simulink model "LCA_feature_mode"  (R2021a)
settings: Solver=VariableStepAuto  StartTime=0.0  StopTime=sim_time  RelTol=1e-3
values from neighbouring files (symbols this model uses):
  L = 4.7    [Pure_Pursiut_Controller_init.m]    (also in Stanley_control_init.m)
  Ld = 10    [Pure_Pursiut_Controller_init.m]
  Vx = 25    [mpc_init.m]
  xRef = refpose(1,:)    [Stanley_control_init.m]    (also in mpc_init.m = refPose(1,:))
  yRef = refpose(2,:)    [Stanley_control_init.m]    (also in mpc_init.m = refPose(2,:) + 2)
undefined symbols (not defined in the file or in its folder): sigbuilder_block
libraries: simulink x2, robotalgslib x1
settings Model: Creator=User  LastModifiedBy=User

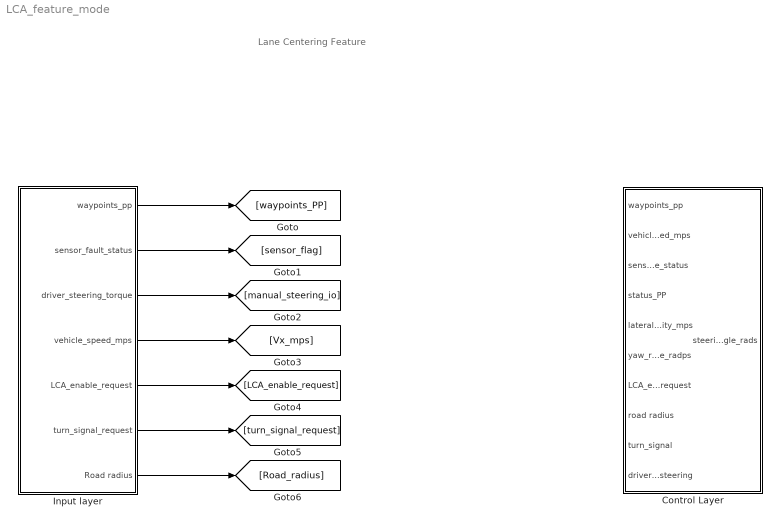
== system LCA_feature_mode ==
  note: Lane Centering Feature
  "\tControl Layer" : Subsystem
  Input layer : Subsystem
  wires:
  Input layer/1(waypoints_pp) -> [waypoints_PP]
  Input layer/2(sensor_fault_status) -> [sensor_flag]
  Input layer/3(driver_steering_torque) -> [manual_steering_io]
  Input layer/4(vehicle_speed_mps) -> [Vx_mps]
  Input layer/5(LCA_enable_request) -> [LCA_enable_request]
  Input layer/6(turn_signal_request) -> [turn_signal_request]
  Input layer/7(Road radius) -> [Road_radius]

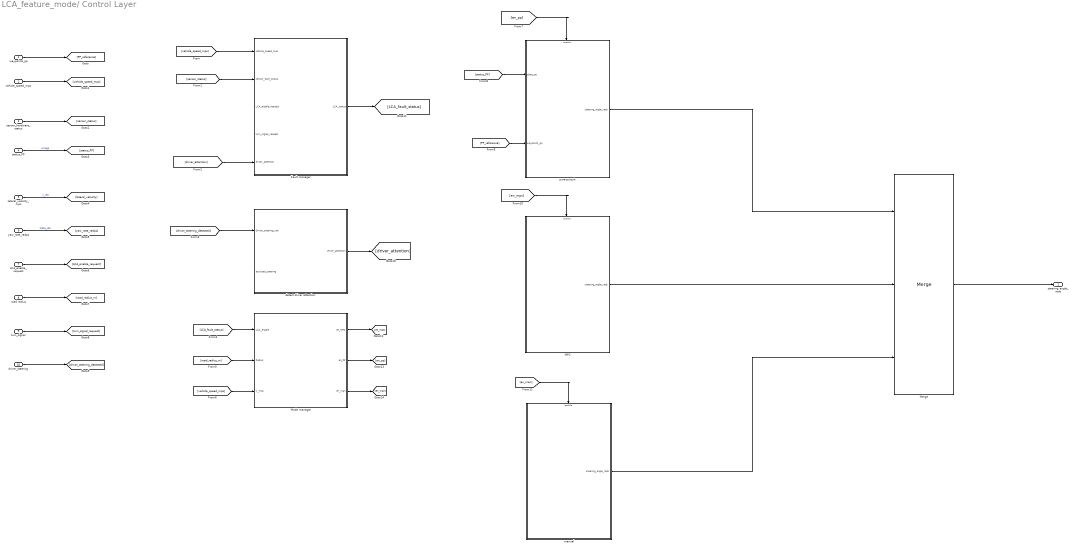
== system LCA_feature_mode/	Control Layer ==
  waypoints_pp : Inport
  vehicle_speed_mps : Inport  Port=2
  sensor_hardware_status : Inport  Port=3
  status_PP : Inport  Port=4
  lateral_velocity_mps : Inport  Port=5
  yaw_rate_radps : Inport  Port=6
  LCA_enable_request : Inport  Port=7
  road radius : Inport  Port=8
  turn_signal : Inport  Port=9
  driver_steering : Inport  Port=10
  Fault manager : Subsystem
  MPC : Subsystem
  Merge : Merge  Inputs=3
  Mode manager : Subsystem
  detect driver attention : Subsystem
  manual : Subsystem
  pure-pursuit : Subsystem
  steering_angle_rads : Outport
  wires:
  waypoints_pp/1 -> [PP_reference]
  vehicle_speed_mps/1 -> [vehicle_speed_mps]
  sensor_hardware_status/1 -> [sensor_status]
  status_PP/1 -> [status_PP]  "omega"
  lateral_velocity_mps/1 -> [lateral_velocity]  "y_dot"
  yaw_rate_radps/1 -> [yaw_rate_radps]  "theta_dot"
  LCA_enable_request/1 -> [LCA_enable_request]
  road radius/1 -> [road_radius_m]
  turn_signal/1 -> [turn_signal_request]
  driver_steering/1 -> [driver_steering_detected]
  [vehicle_speed_mps] -> Fault manager/1(vehicle_speed_mps)
  [sensor_status] -> Fault manager/2(sensor_fault_status)
  detect driver attention/1(driver_attention) -> [driver_attention]
  [driver_attention] -> Fault manager/5("\tdriver_attention")
  [driver_steering_detected] -> detect driver attention/1(Driver_steering_rad)
  Fault manager/1(LCA_status) -> [LCA_fault_status]
  [LCA_fault_status] -> Mode manager/1(LCA_enable)
  [road_radius_m] -> Mode manager/2(Radius)
  [vehicle_speed_mps] -> Mode manager/3(V_mps)
  Mode manager/1(en_MPC) -> [en_mpc]
  Mode manager/2(en_PP) -> [en_pp]
  Mode manager/3(en_man) -> [en_man]
  [en_pp] -> pure-pursuit/Enable
  [status_PP] -> pure-pursuit/1(state_pp)
  [PP_reference] -> pure-pursuit/2(waypoints_pp)
  pure-pursuit/1(steering_angle_rads) -> Merge/1
  MPC/1(steering_angle_rads) -> Merge/2
  [en_mpc] -> MPC/Enable
  [en_man] -> manual/Enable
  manual/1(steering_angle_rads) -> Merge/3
  Merge/1 -> steering_angle_rads/1

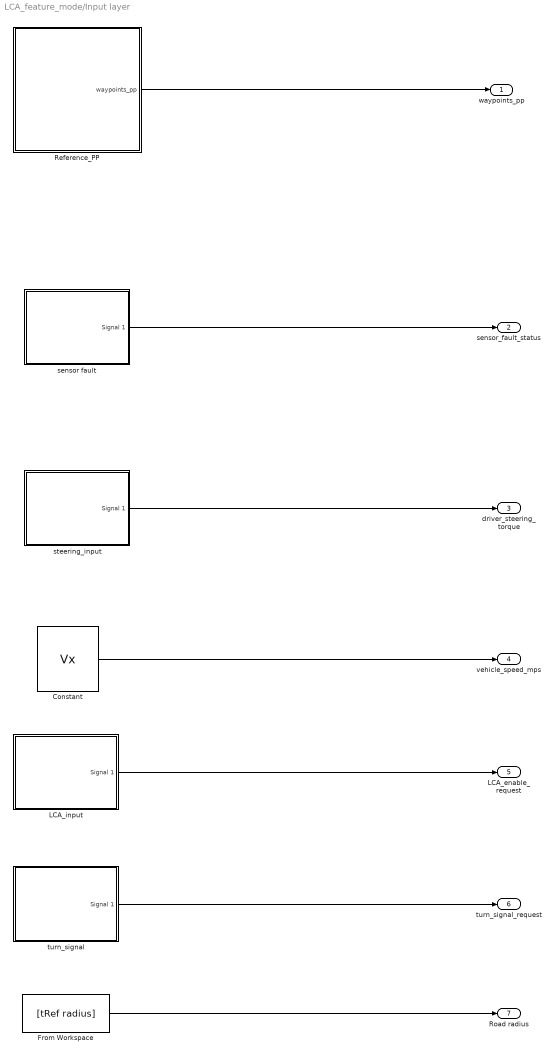
== system LCA_feature_mode/Input layer ==
  Constant : Constant  Value=Vx
  From Workspace : FromWorkspace  VariableName=[tRef radius]  SampleTime=0.1
  LCA_input : Subsystem  Tag=STV Subsys  LoadFcn=sigbuilder_block('load');  StartFcn=sigbuilder_block('start');  StopFcn=sigbuilder_block('stop');  ClipboardFcn=sigbuilder_block('clipboard');  mask(Sigbuilder block){tuvar=[0:10]}
      mask help: Simulink:masks:SigbuilderBlock_MD
      mask init:
      | if ~strcmp(get_param(bdroot(gcbh),'SimulationStatus'),'stopped') tuvar = sigbuilder_block('maskInit'); end
      settings: CopyFcn=sigbuilder_block('copy');  DeleteFcn=sigbuilder_block('delete');  ModelCloseFcn=sigbuilder_block('modelClose');  PreSaveFcn=sigbuilder_block('preSave');  PauseFcn=sigbuilder_block('pause');  ContinueFcn=sigbuilder_block('continue');  NameChangeFcn=sigbuilder_block('namechange');  OpenFcn=sigbuilder_block('open',[309 216.75 550.5 359.25 ]);  CloseFcn=sigbuilder_block('close');
      mask Display: plot(0, 0, 100, 100,[2, 2, 32, 32, 2], [68, 8, 8, 68, 68],[32, 2], [38, 38], [32, 19, 2],[53, 60, 44], [32, 17, 17, 2],[16, 16, 31, 31]);txt = getActiveGroup(gcbh);text(2, 100, txt,'verticalAlignment', 'top');
  Reference_PP : Subsystem
  sensor fault : Subsystem  Tag=STV Subsys  LoadFcn=sigbuilder_block('load');  StartFcn=sigbuilder_block('start');  StopFcn=sigbuilder_block('stop');  ClipboardFcn=sigbuilder_block('clipboard');  mask(Sigbuilder block){tuvar=[0:10]}
      mask help: Simulink:masks:SigbuilderBlock_MD
      mask init:
      | if ~strcmp(get_param(bdroot(gcbh),'SimulationStatus'),'stopped') tuvar = sigbuilder_block('maskInit'); end
      settings: CopyFcn=sigbuilder_block('copy');  DeleteFcn=sigbuilder_block('delete');  ModelCloseFcn=sigbuilder_block('modelClose');  PreSaveFcn=sigbuilder_block('preSave');  PauseFcn=sigbuilder_block('pause');  ContinueFcn=sigbuilder_block('continue');  NameChangeFcn=sigbuilder_block('namechange');  OpenFcn=sigbuilder_block('open',[309 216.75 550.5 359.25 ]);  CloseFcn=sigbuilder_block('close');
      mask Display: plot(0, 0, 100, 100,[2, 2, 32, 32, 2], [68, 8, 8, 68, 68],[32, 2], [38, 38], [32, 19, 2],[53, 60, 44], [32, 17, 17, 2],[16, 16, 31, 31]);txt = getActiveGroup(gcbh);text(2, 100, txt,'verticalAlignment', 'top');
  steering_input : Subsystem  Tag=STV Subsys  LoadFcn=sigbuilder_block('load');  StartFcn=sigbuilder_block('start');  StopFcn=sigbuilder_block('stop');  ClipboardFcn=sigbuilder_block('clipboard');  mask(Sigbuilder block){tuvar=[0:10]}
      mask help: Simulink:masks:SigbuilderBlock_MD
      mask init:
      | if ~strcmp(get_param(bdroot(gcbh),'SimulationStatus'),'stopped') tuvar = sigbuilder_block('maskInit'); end
      settings: CopyFcn=sigbuilder_block('copy');  DeleteFcn=sigbuilder_block('delete');  ModelCloseFcn=sigbuilder_block('modelClose');  PreSaveFcn=sigbuilder_block('preSave');  PauseFcn=sigbuilder_block('pause');  ContinueFcn=sigbuilder_block('continue');  NameChangeFcn=sigbuilder_block('namechange');  OpenFcn=sigbuilder_block('open',[309 216.75 550.5 359.25 ]);  CloseFcn=sigbuilder_block('close');
      mask Display: plot(0, 0, 100, 100,[2, 2, 32, 32, 2], [68, 8, 8, 68, 68],[32, 2], [38, 38], [32, 19, 2],[53, 60, 44], [32, 17, 17, 2],[16, 16, 31, 31]);txt = getActiveGroup(gcbh);text(2, 100, txt,'verticalAlignment', 'top');
  turn_signal : Subsystem  Tag=STV Subsys  LoadFcn=sigbuilder_block('load');  StartFcn=sigbuilder_block('start');  StopFcn=sigbuilder_block('stop');  ClipboardFcn=sigbuilder_block('clipboard');  mask(Sigbuilder block){tuvar=[0:10]}
      mask help: Simulink:masks:SigbuilderBlock_MD
      mask init:
      | if ~strcmp(get_param(bdroot(gcbh),'SimulationStatus'),'stopped') tuvar = sigbuilder_block('maskInit'); end
      settings: CopyFcn=sigbuilder_block('copy');  DeleteFcn=sigbuilder_block('delete');  ModelCloseFcn=sigbuilder_block('modelClose');  PreSaveFcn=sigbuilder_block('preSave');  PauseFcn=sigbuilder_block('pause');  ContinueFcn=sigbuilder_block('continue');  NameChangeFcn=sigbuilder_block('namechange');  OpenFcn=sigbuilder_block('open',[309 216.75 550.5 359.25 ]);  CloseFcn=sigbuilder_block('close');
      mask Display: plot(0, 0, 100, 100,[2, 2, 32, 32, 2], [68, 8, 8, 68, 68],[32, 2], [38, 38], [32, 19, 2],[53, 60, 44], [32, 17, 17, 2],[16, 16, 31, 31]);txt = getActiveGroup(gcbh);text(2, 100, txt,'verticalAlignment', 'top');
  waypoints_pp : Outport
  sensor_fault_status : Outport  Port=2
  driver_steering_torque : Outport  Port=3
  vehicle_speed_mps : Outport  Port=4
  LCA_enable_request : Outport  Port=5
  turn_signal_request : Outport  Port=6
  Road radius : Outport  Port=7
  wires:
  Reference_PP/1(waypoints_pp) -> waypoints_pp/1
  sensor fault/1(Signal 1) -> sensor_fault_status/1
  steering_input/1(Signal 1) -> driver_steering_torque/1
  Constant/1 -> vehicle_speed_mps/1
  LCA_input/1(Signal 1) -> LCA_enable_request/1
  turn_signal/1(Signal 1) -> turn_signal_request/1
  From Workspace/1 -> Road radius/1

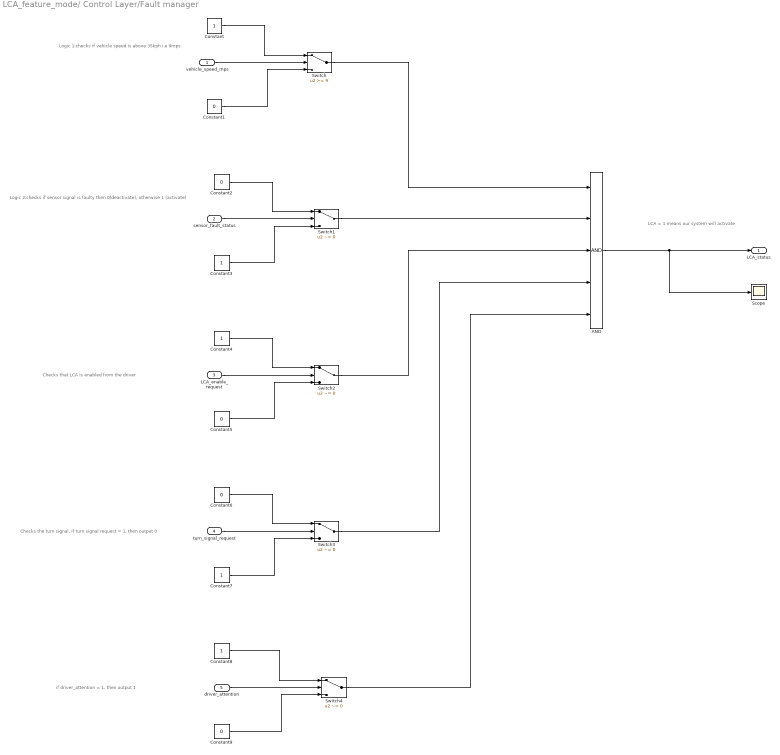
== system LCA_feature_mode/	Control Layer/Fault manager ==
  note: Logic 1:checks if vehicle speed is above 35kph i.e 9mps
  note: Logic 2:checks if sensor signal is faulty then 0(deactivate), otherwise 1 (activate)
  note: Checks that LCA is enabled from the driver
  note: Checks the turn signal. if turn signal request = 1, then output 0
  note: if driver_attention = 1, then output 1
  note: LCA = 1 means our system will activate
  vehicle_speed_mps : Inport
  sensor_fault_status : Inport  Port=2
  "\tLCA_enable_request" : Inport  Port=3
  "\tturn_signal_request" : Inport  Port=4
  "\tdriver_attention" : Inport  Port=5
  AND : Logic  Inputs=5  AllPortsSameDT=off  OutDataTypeStr=boolean
  Constant{,3..4,7..8} (5 alike) : Constant
  Constant{1..2,5..6,9} (5 alike) : Constant  Value=0
  Scope : Scope
  Switch : Switch  Threshold=9
  Switch{1..4} (4 alike) : Switch  Criteria=u2 ~= 0
  LCA_status : Outport
  wires:
  vehicle_speed_mps/1 -> Switch/2
  Constant/1 -> Switch/1
  Constant1/1 -> Switch/3
  Constant3/1 -> Switch1/3
  Constant2/1 -> Switch1/1
  sensor_fault_status/1 -> Switch1/2
  "\tLCA_enable_request"/1 -> Switch2/2
  Constant4/1 -> Switch2/1
  Constant5/1 -> Switch2/3
  Constant7/1 -> Switch3/3
  Constant6/1 -> Switch3/1
  "\tturn_signal_request"/1 -> Switch3/2
  "\tdriver_attention"/1 -> Switch4/2
  Constant8/1 -> Switch4/1
  Constant9/1 -> Switch4/3
  Switch/1 -> AND/1
  Switch1/1 -> AND/2
  Switch2/1 -> AND/3
  Switch3/1 -> AND/4
  Switch4/1 -> AND/5
  AND/1 -> Scope/1, LCA_status/1

== system LCA_feature_mode/	Control Layer/MPC ==
  Enable : EnablePort
  steering_angle_rads : Outport

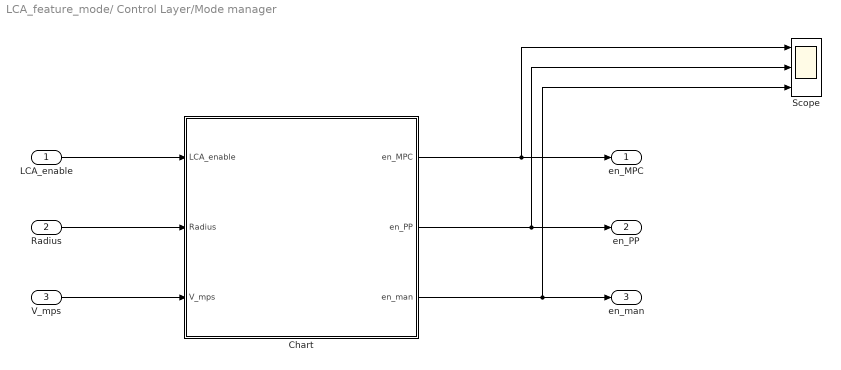
== system LCA_feature_mode/	Control Layer/Mode manager ==
  LCA_enable : Inport
  Radius : Inport  Port=2
  V_mps : Inport  Port=3
  Chart : Stateflow chart  TreatAsAtomicUnit=on
  Scope : Scope  NumInputPorts=3
  en_MPC : Outport
  en_PP : Outport  Port=2
  en_man : Outport  Port=3
  wires:
  LCA_enable/1 -> Chart/1(LCA_enable)
  Radius/1 -> Chart/2(Radius)
  V_mps/1 -> Chart/3(V_mps)
  Chart/1(en_MPC) -> Scope/1, en_MPC/1
  Chart/2(en_PP) -> Scope/2, en_PP/1
  Chart/3(en_man) -> Scope/3, en_man/1

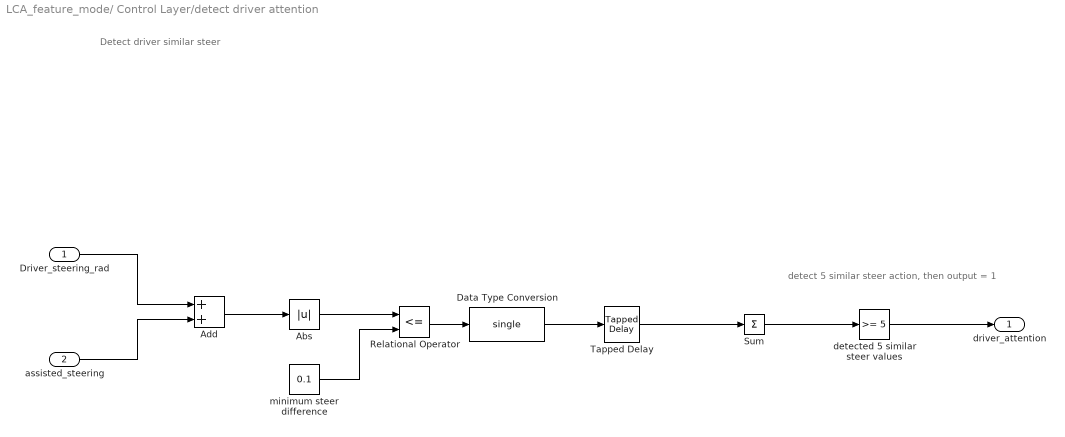
== system LCA_feature_mode/	Control Layer/detect driver attention ==
  note: detect 5 similar steer action, then output = 1
  note: Detect driver similar steer
  Driver_steering_rad : Inport
  assisted_steering : Inport  Port=2
  Abs : Abs
  Add : Sum
  Data Type Conversion : DataTypeConversion  OutDataTypeStr=single
  Relational Operator : RelationalOperator  Operator=<=  OutDataTypeStr=boolean  RndMeth=Simplest
  Sum : Sum  Inputs=+
  Tapped Delay : simulink/Discrete/Tapped Delay  vinit=0.0  samptime=-1  NumDelays=5  DelayOrder=Oldest  includeCurrent=off
  detected 5 similar steer values : simulink/Logic and Bit Operations/Compare To Constant  relop=>=  const=5  OutDataTypeStr=boolean
  minimum steer difference : Constant  Value=0.1
  driver_attention : Outport
  wires:
  Driver_steering_rad/1 -> Add/1
  assisted_steering/1 -> Add/2
  Add/1 -> Abs/1
  Abs/1 -> Relational Operator/1
  minimum steer difference/1 -> Relational Operator/2
  Relational Operator/1 -> Data Type Conversion/1
  Data Type Conversion/1 -> Tapped Delay/1
  Tapped Delay/1 -> Sum/1
  Sum/1 -> detected 5 similar steer values/1
  detected 5 similar steer values/1 -> driver_attention/1

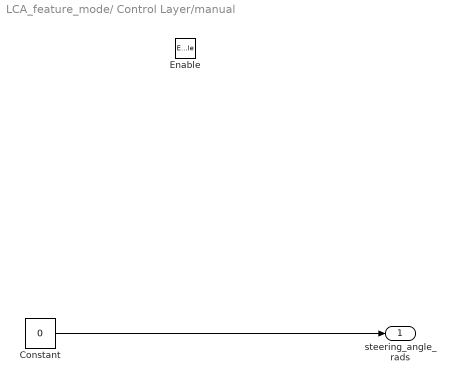
== system LCA_feature_mode/	Control Layer/manual ==
  Enable : EnablePort
  Constant : Constant  Value=0
  steering_angle_rads : Outport
  wires:
  Constant/1 -> steering_angle_rads/1

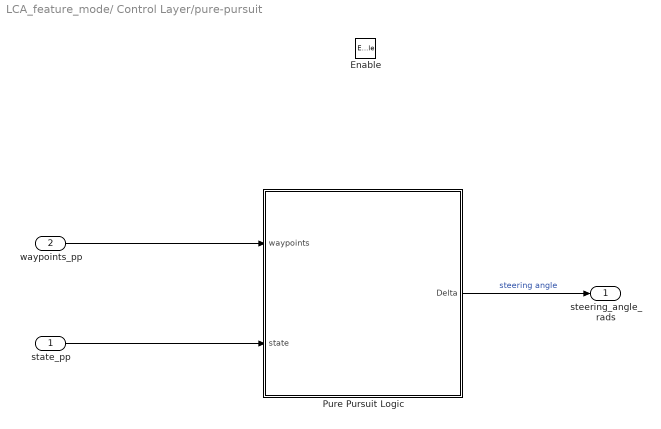
== system LCA_feature_mode/	Control Layer/pure-pursuit ==
  state_pp : Inport
  waypoints_pp : Inport  Port=2
  Enable : EnablePort
  Pure Pursuit Logic : Subsystem
  steering_angle_rads : Outport
  wires:
  state_pp/1 -> Pure Pursuit Logic/2(state)
  waypoints_pp/1 -> Pure Pursuit Logic/1(waypoints)
  Pure Pursuit Logic/1(Delta) -> steering_angle_rads/1  "steering angle"

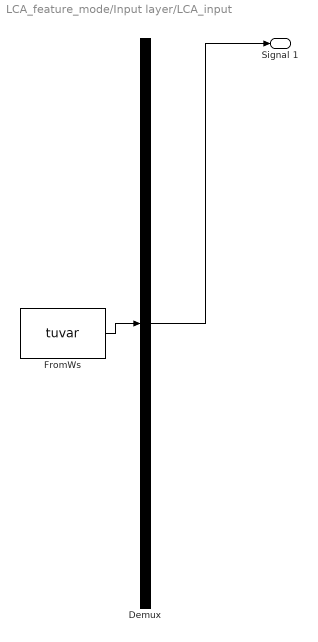
== system LCA_feature_mode/Input layer/LCA_input ==
  Demux : Demux  Tag=STV Demux  Outputs=1
      settings: DisplayOption=none
  FromWs : FromWorkspace  Tag=STV FromWs  VariableName=tuvar
      SigBuilderData=|
      | common.afterFinalStr = 'Extrapolate'
      | common.sampleTime = 0
      | dataSet.timeRange = [0 10]
      | dataSet.name = 'Group 1'
      | sbobj.Groups.Name = 'Group 1'
      | sbobj.Groups.Signals.Name = 'Signal 1'
      | sbobj.Groups.Signals.XData = [0 4 4 6 6 10]
      | sbobj.Groups.Signals.YData = [0 0 1 1 0 0]
  Signal 1 : Outport  Tag=STV Outport
  wires:
  Demux/1 -> Signal 1/1
  FromWs/1 -> Demux/1

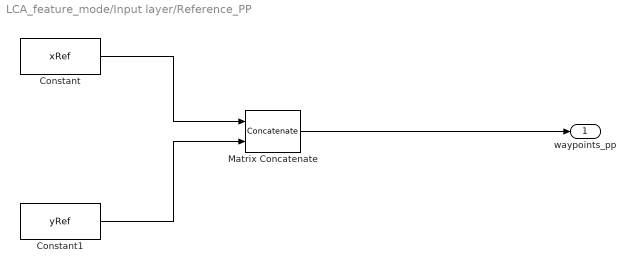
== system LCA_feature_mode/Input layer/Reference_PP ==
  Constant : Constant  Value=xRef  SampleTime=0.1
  Constant1 : Constant  Value=yRef  SampleTime=0.1
  Matrix Concatenate : Concatenate  Mode=Multidimensional array  ConcatenateDimension=2
  waypoints_pp : Outport
  wires:
  Constant/1 -> Matrix Concatenate/1
  Constant1/1 -> Matrix Concatenate/2
  Matrix Concatenate/1 -> waypoints_pp/1

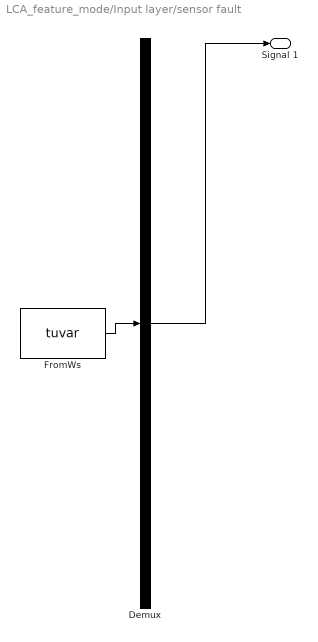
== system LCA_feature_mode/Input layer/sensor fault ==
  Demux : Demux  Tag=STV Demux  Outputs=1
      settings: DisplayOption=none
  FromWs : FromWorkspace  Tag=STV FromWs  VariableName=tuvar
      SigBuilderData=|
      | common.afterFinalStr = 'Extrapolate'
      | common.sampleTime = 0
      | dataSet.timeRange = [0 10]
      | dataSet.name = 'Group 1'
      | sbobj.Groups.Name = 'Group 1'
      | sbobj.Groups.Signals.Name = 'Signal 1'
      | sbobj.Groups.Signals.XData = [0 4 4 6 6 10]
      | sbobj.Groups.Signals.YData = [0 0 1 1 0 0]
  Signal 1 : Outport  Tag=STV Outport
  wires:
  Demux/1 -> Signal 1/1
  FromWs/1 -> Demux/1

== system LCA_feature_mode/Input layer/steering_input ==
  Demux : Demux  Tag=STV Demux  Outputs=1
      settings: DisplayOption=none
  FromWs : FromWorkspace  Tag=STV FromWs  VariableName=tuvar
      SigBuilderData=|
      | common.afterFinalStr = 'Extrapolate'
      | common.sampleTime = 0
      | dataSet.timeRange = [0 10]
      | dataSet.name = 'Group 1'
      | sbobj.Groups.Name = 'Group 1'
      | sbobj.Groups.Signals.Name = 'Signal 1'
      | sbobj.Groups.Signals.XData = [0 4 4 6 6 10]
      | sbobj.Groups.Signals.YData = [0 0 1 1 0 0]
  Signal 1 : Outport  Tag=STV Outport
  wires:
  FromWs/1 -> Demux/1
  Demux/1 -> Signal 1/1

== system LCA_feature_mode/Input layer/turn_signal ==
  Demux : Demux  Tag=STV Demux  Outputs=1
      settings: DisplayOption=none
  FromWs : FromWorkspace  Tag=STV FromWs  VariableName=tuvar
      SigBuilderData=|
      | common.afterFinalStr = 'Extrapolate'
      | common.sampleTime = 0
      | dataSet.timeRange = [0 10]
      | dataSet.name = 'Group 1'
      | sbobj.Groups.Name = 'Group 1'
      | sbobj.Groups.Signals.Name = 'Signal 1'
      | sbobj.Groups.Signals.XData = [0 4 4 6 6 10]
      | sbobj.Groups.Signals.YData = [0 0 1 1 0 0]
  Signal 1 : Outport  Tag=STV Outport
  wires:
  FromWs/1 -> Demux/1
  Demux/1 -> Signal 1/1

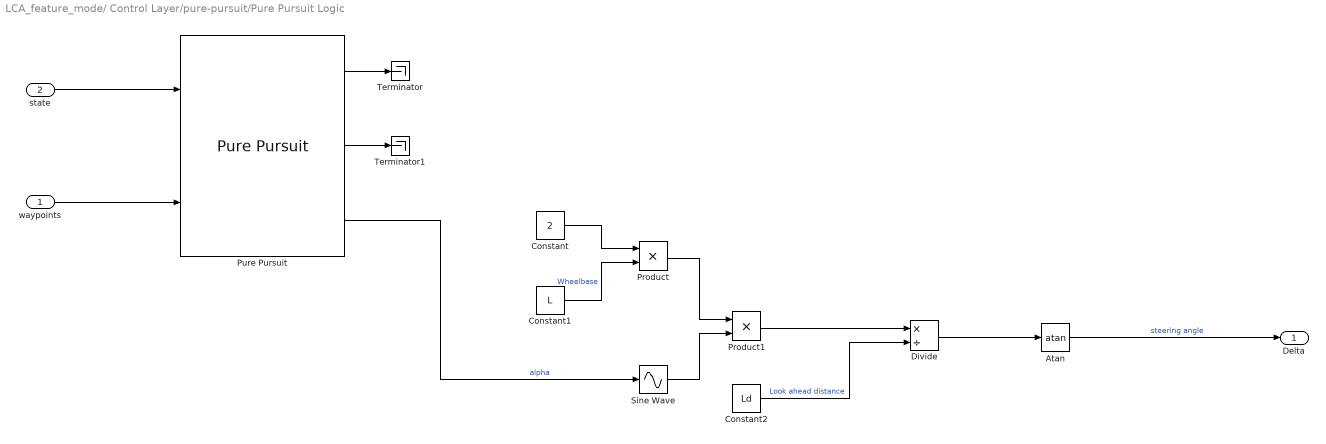
== system LCA_feature_mode/	Control Layer/pure-pursuit/Pure Pursuit Logic ==
  waypoints : Inport
  state : Inport  Port=2
  Atan : Trigonometry  Operator=atan
  Constant : Constant  Value=2
  Constant1 : Constant  Value=L
  Constant2 : Constant  Value=Ld
  Divide : Product  Inputs=*/
  Product : Product
  Product1 : Product
  Pure Pursuit : robotalgslib/Pure Pursuit  DesiredLinearVelocity=Vref  MaxAngularVelocity=1.0  LookaheadDistance=Ld  TargetDirPort=on  SimulateUsing=Code generation
  Sine Wave : Sin  TimeSource=Use external signal  SampleTime=0
  Terminator : Terminator
  Terminator1 : Terminator
  Delta : Outport
  wires:
  Atan/1 -> Delta/1  "steering angle"
  Divide/1 -> Atan/1
  Constant2/1 -> Divide/2  "Look ahead distance"
  Product1/1 -> Divide/1
  Sine Wave/1 -> Product1/2
  Product/1 -> Product1/1
  Constant1/1 -> Product/2  "Wheelbase"
  Constant/1 -> Product/1
  Pure Pursuit/3 -> Sine Wave/1  "alpha"
  Pure Pursuit/2 -> Terminator1/1
  Pure Pursuit/1 -> Terminator/1
  waypoints/1 -> Pure Pursuit/2
  state/1 -> Pure Pursuit/1

== stateflow chart LCA_feature_mode/	Control Layer/Mode manager/Chart ==
  state LCA_off
    entry:en_man = true;
    en_PP = false;
    en_MPC = false;
  state LCA_On
    state PP
      entry:en_man = false;
      en_PP = true;
      en_MPC = false;
    state MPC
      entry:en_man = false;
      en_PP = false;
      en_MPC = true;
    (default) -> PP
    PP -> MPC : [((V_mps > 10) &&(Radius >= 1000)) || ((V_mps > 10) &&(Radius < 1000))]
    MPC -> PP : [((V_mps <= 10) &&(Radius >= 1000)) || ((V_mps <= 10) &&(Radius < 1000)) ]
  (default) -> LCA_off
  LCA_off -> LCA_On : [(LCA_enable) == 1]
  LCA_On -> LCA_off : [(LCA_enable) == 0]
  data: LCA_enable input; Radius input; V_mps input; en_MPC output; en_PP output; en_man output
